simulink model "NMPCLib"  (R2015b)
settings: Solver=VariableStepAuto  StartTime=0.0  StopTime=10.0  RelTol=1e-3
undefined symbols (not defined in the file or in its folder): dU0, U0
settings Model: Creator=stajeddi  LastModifiedBy=stajeddi

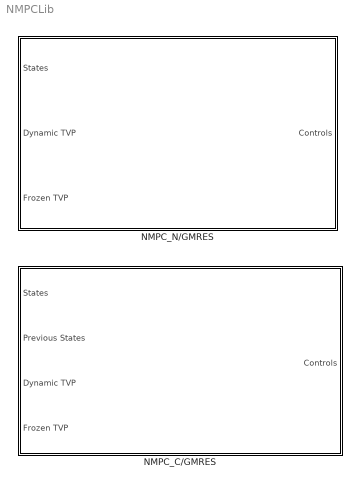
== system NMPCLib ==
  NMPC_C/GMRES : Subsystem
  NMPC_N/GMRES : Subsystem

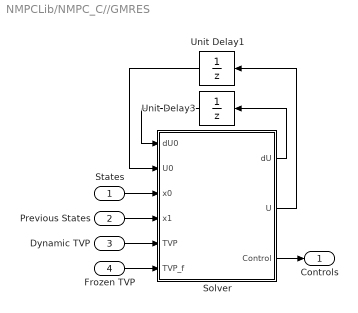
== system NMPCLib/NMPC_C//GMRES ==
  States : Inport
  Previous States : Inport  Port=2
  Dynamic TVP : Inport  Port=3
  Frozen TVP : Inport  Port=4
  Solver : MATLAB Function  TreatAsAtomicUnit=on
  Unit Delay1 : UnitDelay  InitialCondition=U0  SampleTime=-1
  Unit Delay3 : UnitDelay  InitialCondition=dU0  SampleTime=-1
  Controls : Outport
  wires:
  Dynamic TVP/1 -> Solver/5(TVP)
  Unit Delay3/1 -> Solver/1(dU0)
  Solver/1(dU) -> Unit Delay3/1
  Unit Delay1/1 -> Solver/2(U0)
  Solver/2(U) -> Unit Delay1/1
  Solver/3(Control) -> Controls/1
  Frozen TVP/1 -> Solver/6(TVP_f)
  States/1 -> Solver/3(x0)
  Previous States/1 -> Solver/4(x1)

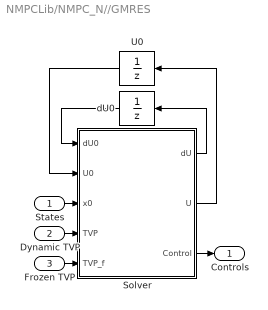
== system NMPCLib/NMPC_N//GMRES ==
  States : Inport
  Dynamic TVP : Inport  Port=2
  Frozen TVP : Inport  Port=3
  Solver : MATLAB Function  TreatAsAtomicUnit=on
  U0 : UnitDelay  InitialCondition=U0  SampleTime=-1
  dU0 : UnitDelay  InitialCondition=dU0  SampleTime=-1
  Controls : Outport
  wires:
  States/1 -> Solver/3(x0)
  Frozen TVP/1 -> Solver/5(TVP_f)
  Solver/3(Control) -> Controls/1
  Solver/2(U) -> U0/1
  U0/1 -> Solver/2(U0)
  Solver/1(dU) -> dU0/1
  dU0/1 -> Solver/1(dU0)
  Dynamic TVP/1 -> Solver/4(TVP)

== matlab function NMPCLib/NMPC_C//GMRES/Solver ==
  data: dU0 input; dU output; U0 input; x0 input; x1 input; TVP input; U output; Control output; TVP_f input
%% Continuation/GMRES  Continuation/GMRES Continuation/GMRES
function [dU,U,Control] = NMPCBlock(dU0,U0,x0,x1,TVP,TVP_f)
[dU,U,Control] = NMPC(dU0,U0,x0,x1,TVP,TVP_f);

== matlab function NMPCLib/NMPC_N//GMRES/Solver ==
  data: dU0 input; dU output; U0 input; x0 input; TVP input; U output; Control output; TVP_f input
%% NGMRES  NGMRES NGMRES
function [dU,U,Control] = NMPCBlock(dU0,U0,x0,TVP,TVP_f)
[dU,U,Control]=NMPC(dU0,U0,x0,TVP,TVP_f);
